simulink model "esercitazione_8_sistema_sim"  (R2022a)
settings: Solver=ode45  StartTime=0.0  StopTime=100  RelTol=1e-3  EnableMultiTasking=on
settings Model: Creator=claudio  LastModifiedBy=Stefano
settings SolverCC: AlgebraicLoopSolver=TrustRegion
settings DataIOCC: LimitDataPoints=on  SaveFormat=Array  ReturnWorkspaceOutputs=off
settings OptimizationCC: LifeSpan=inf
settings DebuggingCC: SolverPrmCheckMsg=warning  UnconnectedInputMsg=warning  UnconnectedOutputMsg=warning  UnconnectedLineMsg=warning  SFUnexpectedBacktrackingDiag=warning  SFNoUnconditionalDefaultTransitionDiag=warning  SFExecutionAtInitializationDiag=none  SFMachineParentedDataDiag=warning  ArithmeticOperatorsInVariantConditions=warning
settings HardwareCC: ProdBitPerPointer=32  ProdBitPerSizeT=32  ProdBitPerPtrDiffT=32  ProdLargestAtomicFloat=None  ProdIntDivRoundTo=Undefined  ProdEndianess=Unspecified  ProdWordSize=32  ProdHWDeviceType=32-bit Generic
settings ModelReferenceCC: PropagateSignalLabelsOutOfModel=off
settings SFSimCC: SimUseLocalCustomCode=off  CustomCodeUndefinedFunction=UseInterfaceOnly
settings RTWCC: RTWUseLocalCustomCode=off
settings CodeAppCC: StateflowObjectComments=on
settings GRTTargetCC: TargetLangStandard=C89/C90 (ANSI)
settings ConfigComp: CovMetricSettings=dw  CovSaveCumulativeToWorkspaceVar=on  CovSaveSingleToWorkspaceVar=on  CovExternalEMLEnable=off  CovSFcnEnable=off

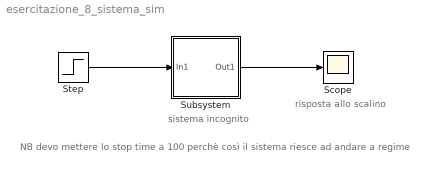
== system esercitazione_8_sistema_sim ==
  note: NB devo mettere lo stop time a 100 perchè così il sistema riesce ad andare a regime
  note: sistema incognito
  note: risposta allo scalino
  Scope : Scope
  Step : Step  Time=0  SampleTime=0
  Subsystem : Subsystem
  wires:
  Step/1 -> Subsystem/1(In1)
  Subsystem/1(Out1) -> Scope/1

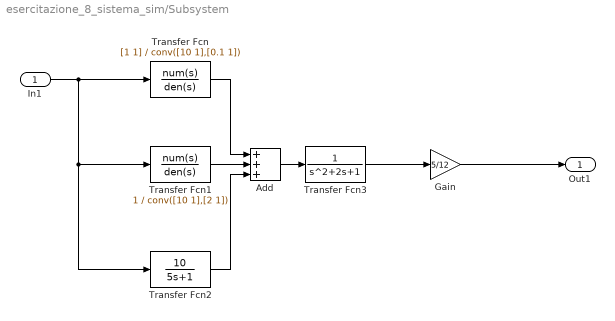
== system esercitazione_8_sistema_sim/Subsystem ==
  In1 : Inport
  Add : Sum  Inputs=+++
  Gain : Gain  Gain=5/12
  Transfer Fcn : TransferFcn  Numerator=[1 1]  Denominator=conv([10 1],[0.1 1])
  Transfer Fcn1 : TransferFcn  Numerator=1  Denominator=conv([10 1],[2 1])
  Transfer Fcn2 : TransferFcn  Numerator=10  Denominator=[5 1]
  Transfer Fcn3 : TransferFcn  Numerator=1
  Out1 : Outport
  wires:
  In1/1 -> Transfer Fcn2/1, Transfer Fcn1/1, Transfer Fcn/1
  Transfer Fcn1/1 -> Add/2
  Transfer Fcn/1 -> Add/1
  Add/1 -> Transfer Fcn3/1
  Transfer Fcn2/1 -> Add/3
  Transfer Fcn3/1 -> Gain/1
  Gain/1 -> Out1/1
